simulink model "boat_model_and_controller2020lqi"  (R2021a)
settings: Solver=VariableStepAuto  StartTime=0.0  StopTime=10  FixedStep=0.01  RelTol=1e-3
undefined symbols (not defined in the file): DiscIntNeverNeededParam, Eff, FF_L, FF_R, initial_P, initial_Pitch, initial_Q, initial_R, initial_ROLL, initial_uspeed, initial_vspeed, initial_wspeed, initial_YAW, initial_Z, Kih, Kir, rear_alfas, T, uncertainty
libraries: simulink x7, simulink_extras x3, dspsrcs4 x1, pid_lib x1
(part 2 of 3)

== matlab function boat_model_and_controller2020lqi/BOAT/model_equations ==
  data: u_dot output; v_dot output; w_dot output; p_dot output; q_dot output; r_dot output; Act_front_left input; Act_front_right input; Act_rear input; Rpms_motor input; Rudder input; u input; v input; w input; p input; qq input; r input; Pitch input; Roll input; Yaw input; z input; Torque output; Rpms_motor output; Lift_Coluna output; Lift_Strut_right output; D_total_strut_right output; drag_col output; bb output; kstrut_left output; kcoluna output; uncertainty input
function [u_dot,v_dot,w_dot,p_dot,q_dot,r_dot,Torque,Rpms_motor,Lift_Coluna,Lift_Strut_right,D_total_strut_right,drag_col,bb,kstrut_left,kcoluna] = model_equations(Act_front_left,Act_front_right,Act_rear,Rpms_motor,Rudder,u,v,w,p,qq,r,Pitch,Roll,Yaw,z,uncertainty)

%%%%%%%%%%%%%%%%%%%%%%%%%%%%%%%%%%%%%%%%%%%%%%%%%SS
%%%%%%%%%%%%%%%% constants %%%%%%%%%%%%%%%%%%%%%%
%%%%%%%%%%%%%%%%%%%%%%%%%%%%%%%%%%%%%%%%%%%%%%%%%
pi=3.14159265358979;
g = 9.81; %gravity (m/s^2)
rho= 1025.00; % Densidade de àgua(kg/m^3)   <-I
mu= 1.14E-3; % Coef. Viscosidade Dinâmica para calular Reynolds(Pa*s)   <-I
m = 180*uncertainty(15); %Weight of boat (Kg) <-I
dist_cm_Us_x = 3.150*uncertainty(16);   %distância ultrassom ao cm
dist_struts_Us_x = 1.850*uncertainty(17);
dist_col_Us_x = 5.520*uncertainty(18);
dy_front = 1.2/2*uncertainty(19); %front foils' y distance divided by 2
dist_x_rear = 2.367*uncertainty(20);
dist_x_front = 1.30156*uncertainty(21);
dist_z_rear = 1.05*uncertainty(22); %ambas desde o CM (z também se mede desde o ultrassom)
dist_z_front = 0.85*uncertainty(23);
coluna_exposta = 0.776*uncertainty(24);
z_cm_sem_roll = cosd(Pitch)*z+tand(Pitch)*dist_cm_Us_x;
z_cm = z_cm_sem_roll/cosd(Roll);
z_struts_sem_roll = z+dist_struts_Us_x*tand(Pitch);
z_col_sem_roll = z+dist_col_Us_x*tand(Pitch); %perpendicular à água no roll
z_strut_left = z_struts_sem_roll - tand(Roll)*dy_front;
z_strut_right = z_struts_sem_roll + tand(Roll)*dy_front;
hf_left = dist_z_front +z_strut_left;
hf_right = dist_z_front+z_strut_right;
hr = dist_z_rear + z_col_sem_roll;

if hr > coluna_exposta
    hr = coluna_exposta;
end
if hf_left > dist_z_front
    hf_left = dist_z_front;
end
if hf_right > dist_z_front
    hf_right = dist_z_front;
end
Iyy = 503*uncertainty(11);        % boat's moment of inertia in kg.m^2 for pitch
Ixx = 31*uncertainty(12);          % moment of inertia for roll
Izz = 300*uncertainty(13);
Ixz = 16.5*uncertainty(14);

%angle of attack
aa = atand(w/u);
bb = asind(v/sqrt(u^2+v^2));
alfa_front_left = Act_front_left + aa;
alfa_front_right = Act_front_right + aa;
alfa_rear = Act_rear + aa;
speed = sqrt(u^2+v^2+w^2);

%%%%%%%%%%%%%%%%%%%%%%%%%%%%%%%%%%%%%%%%%%%%%%%%%
%%%%%%%%%%%%%%%% Geometry %%%%%%%%%%%%%%%%%%%%%%%
%%%%%%%%%%%%%%%%%%%%%%%%%%%%%%%%%%%%%%%%%%%%%%%%%
a = 1;
%Geometria foil frente(x2)
cff=0.08; % Corda foil frente(m)
tff=0.12; % Espessura maxima perfil foil frente (n63412: t=0.12c)
bff=0.8; % Envergadura foil frente (m)
Sff=1.05*pi*bff*cff/4*a; %Area planform foil frente (m^2) --  0.04773 valor dos foils atuais
SAff=Sff*2; % Area superficie foil frente (assumir 2x planform area) (m^2)
ARf=bff^2/Sff; %Aspect ratio foil frente
cordfun = @(x) cff.^2 .*(x-(x.^3/(bff/2).^2)/3);
MACf =  2/Sff*(cordfun(bff/2)-cordfun(0));
cff=MACf;
k2f_left = (16*(hf_left/MACf)^2+2)/(16*(hf_left/MACf)^2+1);
k2f_right = (16*(hf_right/MACf)^2+2)/(16*(hf_right/MACf)^2+1);

%Geometria foil trás
cft=0.08; % Corda foil trás (m)
tft=0.12; % Espessura maxima foil tras (n63412: t=0.12c)
bft=0.8; % Envergadura foil tras (m)
Sft=1.05*pi*bft*cft/4*a; %Area planform foil tras (m^2) --- 0.04584 valor dos foils atuais
SAft=Sft*2; % Area superficie foil tras (assumir 2x planform area) (m^2)
ARt=bft^2/Sft; %Aspect ratio foil tras
cordfun = @(x) cft.^2 .*(x-(x.^3/(bft/2).^2)/3);
MACt = 2/Sft*(cordfun(bft/2)-cordfun(0));
cft=MACt;
k2t = (16*(hr/MACt)^2+2)/(16*(hr/MACf)^2+1);
%Geometria Struts
cs= 0.13; % Corda strut (m)
ts=0.12; % Espessura maxima perfil strut (n0012: t=0.12c)
Ss_left=cs*hf_left; %area planform strut (m^2)
SAs_left=2*Ss_left; % Area superficie strut (SOLIDWORKS) (m^2)
substrut_left=hf_left/cs; %aspect ratio da seccao submergida strut
Ss_right=cs*hf_right; %area planform strut (m^2)
SAs_right=2*Ss_right; % Area superficie strut (SOLIDWORKS) (m^2)
substrut_right=hf_right/cs; %aspect ratio da seccao submergida strut


%Geometria Coluna
cc=0.17; % corda coluna (m)
tc=0.18; % Espessura maxima perfil coluna (n0012: t=0.12c)
Sc=cc*hr; %area planform coluna (m^2)
SAc=2*Sc; % Area superficie coluna (m^2)
subcol=hr/cc; %aspect ratio da seccao submergida coluna


%%%%%%%%%%%%%%%%%%%%%%%%%%%%%%%%%%%%%%%%%%%%%%%%%
%%%%%%%%%%%%%%%% pre-calculations %%%%%%%%%%%%%%%
%%%%%%%%%%%%%%%%%%%%%%%%%%%%%%%%%%%%%%%%%%%%%%%%%

q = 0.5*rho*speed^2;%Pressao dinamica (Kg m^-1 s^-2)

Tff=cff*tff; % Thicknes front foil= chord*t
Tft=cft*tft;% Thicknes rear foil= chord*t
Ts=cs*ts; % Thicknes strut= chord*t
Tc=cc*tc;% Thicknes coluna= chord*t

Reff=(rho)*(speed)*(cff)/(mu); %Num Reynolds foil frente
Reft=(rho)*(speed)*(cft)/(mu); %Num Reynold foil tras
Restrut=(rho)*(speed)*(cs)/(mu); %Num Reynolds strut
Recol=(rho)*(speed)*(cc)/(mu); %Num Reynolds coluna

%determining cd of the foils, struts and prop column

%strut pressure drag. Column assumed to have same pressure drag as
%strut

p00 =     0.01162;
p10 =  -7.938e-07;
p01 =  -5.664e-05;
p20 =   0.0001378;
p11 =   3.735e-08;
p02 =   1.241e-07;
p30 =  -1.257e-07;
p21 =   -4.13e-07;
p12 =  -9.269e-11;
p03 =  -1.231e-10;
p40 =   1.604e-06;
p31 =    4.88e-10;
p22 =   4.056e-10;
p13 =   6.432e-14;
p04 =   5.515e-14;
p50 =  -1.201e-09;
p41 =  -1.096e-09;
p32 =   -1.95e-13;
p23 =   -1.04e-13;
p14 =   -1.36e-17;
p05 =   -9.13e-18;

cdpstrut =@(x,y) p00 + p10*x + p01*y + p20*x^2 + p11*x*y + p02*y^2 + p30*x^3 + p21*x^2*y ...
    + p12*x*y^2 + p03*y^3 + p40*x^4 + p31*x^3*y + p22*x^2*y^2 ...
    + p13*x*y^3 + p04*y^4 + p50*x^5 + p41*x^4*y + p32*x^3*y^2 ...
    + p23*x^2*y^3 + p14*x*y^4 + p05*y^5;

CDp_s = cdpstrut(bb,Restrut/1000)*uncertainty(1);
CDp_c = cdpstrut(bb+Rudder,Recol/1000)*uncertainty(2);

%determining coefficient of lift of the foils for a set angle of attack
p00 =     0.04647;
p10 =      0.1369;
p01 =    0.001502;
p20 =   0.0005872;
p11 =  -0.0001138;
p02 =  -2.794e-06;
p30 =  -0.0007229;
p21 =  -2.662e-07;
p12 =   1.545e-07;
p03 =   2.428e-09;
p40 =   1.647e-05;
p31 =   6.574e-07;
p22 =  -3.892e-09;
p13 =  -7.221e-11;
p04 =  -9.966e-13;
p50 =  -6.807e-08;
p41 =  -2.534e-09;
p32 =  -2.657e-10;
p23 =   2.267e-12;
p14 =   9.751e-15;
p05 =   1.555e-16;

clf = @(x,y) p00 + p10*x + p01*y + p20*x^2 + p11*x*y + p02*y^2 + p30*x^3 + p21*x^2*y ...
    + p12*x*y^2 + p03*y^3 + p40*x^4 + p31*x^3*y + p22*x^2*y^2 ...
    + p13*x*y^3 + p04*y^4 + p50*x^5 + p41*x^4*y + p32*x^3*y^2 ...
    + p23*x^2*y^3 + p14*x*y^4 + p05*y^5;

clff_left = clf(alfa_front_left,Reff/1000)*uncertainty(3);
clff_right = clf(alfa_front_right,Reff/1000)*uncertainty(3);
clrf = clf(alfa_rear,Reft/1000)*uncertainty(4);
CL_f_3D_left =clff_left*(ARf/(ARf+2))*k2f_left;
CL_f_3D_right =clff_right*(ARf/(ARf+2))*k2f_right;
CL_t_3D =clrf*(ARt/(ARt+2))*k2t;

%determining coefficient of pressure drag of the foils
p00 =     0.01465;
p10 =  -0.0003439;
p01 =  -5.436e-05;
p20 =  -0.0002518;
p11 =   1.629e-06;
p02 =   8.999e-08;
p30 =   1.962e-05;
p21 =   5.111e-07;
p12 =  -2.115e-09;
p03 =  -7.446e-11;
p40 =    6.85e-06;
p31 =  -4.153e-08;
p22 =  -2.604e-10;
p13 =   1.213e-12;
p04 =   3.002e-14;
p50 =  -3.572e-07;
p41 =  -2.379e-09;
p32 =   1.914e-11;
p23 =   3.918e-14;
p14 =  -2.599e-16;
p05 =  -4.682e-18;

cdpf = @(x,y) p00 + p10*x + p01*y + p20*x^2 + p11*x*y + p02*y^2 + p30*x^3 + p21*x^2*y ...
    + p12*x*y^2 + p03*y^3 + p40*x^4 + p31*x^3*y + p22*x^2*y^2 ...
    + p13*x*y^3 + p04*y^4 + p50*x^5 + p41*x^4*y + p32*x^3*y^2 ...
    + p23*x^2*y^3 + p14*x*y^4 + p05*y^5;

cdp_ff_left = cdpf(alfa_front_left,Reff/1000)*uncertainty(5);
cdp_ff_right = cdpf(alfa_front_right,Reff/1000)*uncertainty(5);
cdp_ft = cdpf(alfa_rear,Reft/1000)*uncertainty(6);

%%%%%%%%%%%%%%%%%%%%%%%%%%%%%%%%%%%%%%%%%%%%%%%%%
%%%%%%%%%%%% boat model equations %%%%%%%%%%%%%%%
%%%%%%%%%%%%%%%%%%%%%%%%%%%%%%%%%%%%%%%%%%%%%%%%%

%Lift (XFRL5)
lift_front_left=(CL_f_3D_left)*q*Sff;
lift_front_right=(CL_f_3D_right)*q*Sff;
lift_rear=(CL_t_3D)*q*Sft;

kstrut_left=1/(13+(13/(substrut_left)^2)+(26/(substrut_left)))*uncertainty(7); % coeficiente de lift que toma em conta a aspect ratio da seccao submergida da strut
kstrut_right=1/(13+(13/(substrut_right)^2)+(26/(substrut_right)))*uncertainty(7); % coeficiente de lift que toma em conta a aspect ratio da seccao submergida da strut
kcoluna=1/(13+(13/(subcol)^2)+(26/(subcol)))*uncertainty(8); % coeficiente de lift que toma em conta a aspect ratio da seccao submergida da coluna
Lift_Strut_left = -1/2*rho*(speed^2)*Ss_left*kstrut_left*bb;
Lift_Strut_right = -1/2*rho*(speed^2)*Ss_right*kstrut_right*bb;
Lift_Coluna = -1/2*rho*(speed^2)*Sc*kcoluna*(bb+Rudder);
bb_Trans_sup = 12;
bb_Trans_inf = 15;

if bb>bb_Trans_sup || bb<-bb_Trans_sup % condicão de ventilacão da strut
    Lift_Strut_Trans_sup_left = -1/2*rho*(speed^2)*Ss_left*kstrut_left*bb_Trans_sup*bb/abs(bb);
    Lift_Strut_Trans_sup_right = -1/2*rho*(speed^2)*Ss_right*kstrut_right*bb_Trans_sup*bb/abs(bb);
    Lift_Strut_Trans_inf_left = -1/2*rho*(speed^2)*Ss_left*(kstrut_left*bb_Trans_inf*bb/abs(bb)-kstrut_left*9*(bb/abs(bb))*abs(1-abs(1/bb_Trans_inf)));
    Lift_Strut_Trans_inf_right = -1/2*rho*(speed^2)*Ss_right*(kstrut_right*bb_Trans_inf*bb/abs(bb)-kstrut_right*9*(bb/abs(bb))*abs(1-abs(1/bb_Trans_inf)));
    Lift_Strut_left = Lift_Strut_Trans_sup_left+(Lift_Strut_Trans_inf_left-Lift_Strut_Trans_sup_left)/(bb_Trans_inf*bb/abs(bb)-bb_Trans_sup*bb/abs(bb))*(bb-bb_Trans_sup*bb/abs(bb));
    Lift_Strut_right = Lift_Strut_Trans_sup_right+(Lift_Strut_Trans_inf_right-Lift_Strut_Trans_sup_right)/(bb_Trans_inf*bb/abs(bb)-bb_Trans_sup*bb/abs(bb))*(bb-bb_Trans_sup*bb/abs(bb));
    if bb>bb_Trans_inf || bb<-bb_Trans_inf
        Lift_Strut_left = -1/2*rho*(speed^2)*Ss_left*(kstrut_left*bb-kstrut_left*9*(bb/abs(bb))*abs(1-abs(1/bb)));
        Lift_Strut_right = -1/2*rho*(speed^2)*Ss_right*(kstrut_right*bb-kstrut_right*9*(bb/abs(bb))*abs(1-abs(1/bb)));
    end
end
if (bb+Rudder)>bb_Trans_sup || (bb+Rudder)<-bb_Trans_sup
    Lift_Coluna = -1/2*rho*speed^2*Sc*(kcoluna*(bb+Rudder)-kcoluna*9*(bb+Rudder)/abs(bb+Rudder));
end

%Induced Drag (XFLR5)
e=1; %oswald efficiency factor (assumir 1 para dist. lift puramente eliptica)
C_Dind_ff_left=(CL_f_3D_left)^2/(pi*e*(ARf)); % Coef Drag Induzido
C_Dind_ff_right=(CL_f_3D_right)^2/(pi*e*(ARf)); % Coef Drag Induzido
C_Dind_rf=(CL_t_3D)^2/(pi*e*(ARt));
D_induced_ff_left=(C_Dind_ff_left)*q*(Sff); %Drag induzido (N)
D_induced_ff_right=(C_Dind_ff_right)*q*(Sff); %Drag induzido (N)
D_induced_rf=(C_Dind_rf)*q*(Sft); %Drag induzido (N)

% Skin Friction Drag

Re_crit=500000;  %Como Rule Of Thumb, assume-se que a transição se dá pontualemente a Re=500 000- Anderson's Fundamentals of Aerodynamics (pg 903)
x_crit=Re_crit*mu/(rho*speed); %calcula o ponto onde se dá a transição na asa retângular
%x_c_crit_n63412=; %  <-M
%x_c_crit_n0012=0.3; %     <-M
%VARIAVEIS DE INPUT VAZIAS PARA FORÇAR A
%TRANSIÇAO NUM PONTO QUE NAO RE 500 000

%Foils frente

C_skf_ff_lam=1.328/(Re_crit)^0.5; %Coef skin friction esc laminar- Hoerner’s Fluid-Dynamic Drag (pg 2-5)-Foil frente
S_ff_lam=Sff*x_crit; %Area de escoamento laminar- corresponde a zona 1-lam
D_skf_ff_lam=q*C_skf_ff_lam*S_ff_lam; %Drag skf foil frente_flat plate_zona 1-lam
C_skf_ff_tur_12=0.455/(log10(Reff)^2.58); %Coef skin friction esc turbulento- Hoerner’s Fluid-Dynamic Drag (pg 2-5)-fim zona 2-tur
C_skf_ff_tur_1=0.455/(log10(Re_crit)^2.58); %coef skf ff esc turbulento- fim zona 1-trans
D_skf_ff_tur_12=q*Sff*C_skf_ff_tur_12; %drag skf ff_flat plate_esc turbulento-fim zona 2-tur
D_skf_ff_tur_1=q*S_ff_lam*C_skf_ff_tur_1;%drag skf ff_flat plate_esc turbulento- fim zona 1-trans
D_skf_ff_tur=D_skf_ff_tur_12-D_skf_ff_tur_1;%drag skf ff_flat plate_esc turbulento total
D_skf_ff_tot_1=D_skf_ff_lam +D_skf_ff_tur; %drag skf ff_flat plate_total
CD_skf_ff=D_skf_ff_tot_1/(q*Sff); %coeficiente de drag de skin friction ff final
D_ffskf=1/2*(CD_skf_ff)*(rho)*(speed)^2*(SAff); %Drag de skin friction final ff


%Foil Tras
C_skf_ft_lam=1.328/(Re_crit)^0.5;%Coef skin friction esc laminar- Hoerner’s Fluid-Dynamic Drag (pg 2-5)-Foil tras
S_ft_lam=Sft*x_crit; %Area de escoamento laminar- corresponde a zona 1-lam
D_skf_ft_lam=q*C_skf_ft_lam*S_ft_lam;%Drag skf foil tras_flat plate_zona 1-lam
C_skf_ft_tur_12=0.455/(log10(Reff)^2.58); %Coef skin friction esc turbulento- Hoerner’s Fluid-Dynamic Drag (pg 2-5)-fim zona 2-tur
C_skf_ft_tur_1=0.455/(log10(Re_crit)^2.58); %coef skf ft esc turbulento- fim zona 1-trans
D_skf_ft_tur_12=q*Sft*C_skf_ft_tur_12;%drag skf ft_flat plate_esc turbulento-fim zona 2-tur
D_skf_ft_tur_1=q*S_ft_lam*C_skf_ft_tur_1;%drag skf ft_flat plate_esc turbulento- fim zona 1-trans
D_skf_ft_tur=D_skf_ft_tur_12-D_skf_ft_tur_1;%drag skf ft_flat plate_esc turbulento total
D_skf_ft_tot_1=D_skf_ft_lam +D_skf_ft_tur; %drag skf ft_flat plate_total
CD_skf_ft=D_skf_ft_tot_1/(q*Sft);%coeficiente de drag de skin friction ft final
D_ftskt=1/2*(CD_skf_ft)*(rho)*(speed)^2*(SAft);%Drag de skin friction final ft



%Strut Esquerda
C_skf_s_lam=1.328/(Re_crit)^0.5;%Coef skin friction esc laminar- Hoerner’s Fluid-Dynamic Drag (pg 2-5)-strut
S_s_lam_left=Ss_left*x_crit; %Area de escoamento laminar- corresponde a zona 1-lam
D_skf_s_lam_left=q*C_skf_s_lam*S_s_lam_left;%Drag skf strut_flat plate_zona 1-lam
C_skf_s_tur_12=0.455/(log10(Restrut)^2.58);%Coef skin friction esc turbulento- Hoerner’s Fluid-Dynamic Drag (pg 2-5)-fim zona 2-tur
C_skf_s_tur_1=0.455/(log10(Re_crit)^2.58);%coef skf s esc turbulento- fim zona 1-trans
D_skf_s_tur_12_left=q*Ss_left*C_skf_s_tur_12;%drag skf s_flat plate_esc turbulento-fim zona 2-tur
D_skf_s_tur_1_left=q*S_s_lam_left*C_skf_s_tur_1;%drag skf s_flat plate_esc turbulento- fim zona 1-trans
D_skf_s_tur_left=D_skf_s_tur_12_left-D_skf_s_tur_1_left; %drag skf s_flat plate_esc turbulento total
D_skf_s_tot_1_left=D_skf_s_lam_left +D_skf_s_tur_left; %drag skf s_flat plate_total
CD_skf_s_left=D_skf_s_tot_1_left/(q*Ss_left);%coeficiente de drag de skin friction s final
D_strutskf_left=1/2*(CD_skf_s_left)*(rho)*(speed)^2*(SAs_left);%Drag de skin friction final strut

%Strut Direita
C_skf_s_lam=1.328/(Re_crit)^0.5;%Coef skin friction esc laminar- Hoerner’s Fluid-Dynamic Drag (pg 2-5)-strut
S_s_lam_right=Ss_right*x_crit; %Area de escoamento laminar- corresponde a zona 1-lam
D_skf_s_lam_right=q*C_skf_s_lam*S_s_lam_right;%Drag skf strut_flat plate_zona 1-lam
C_skf_s_tur_12=0.455/(log10(Restrut)^2.58);%Coef skin friction esc turbulento- Hoerner’s Fluid-Dynamic Drag (pg 2-5)-fim zona 2-tur
C_skf_s_tur_1=0.455/(log10(Re_crit)^2.58);%coef skf s esc turbulento- fim zona 1-trans
D_skf_s_tur_12_right=q*Ss_right*C_skf_s_tur_12;%drag skf s_flat plate_esc turbulento-fim zona 2-tur
D_skf_s_tur_1_right=q*S_s_lam_right*C_skf_s_tur_1;%drag skf s_flat plate_esc turbulento- fim zona 1-trans
D_skf_s_tur_right=D_skf_s_tur_12_right-D_skf_s_tur_1_right; %drag skf s_flat plate_esc turbulento total
D_skf_s_tot_1_right=D_skf_s_lam_right +D_skf_s_tur_right; %drag skf s_flat plate_total
CD_skf_s_right=D_skf_s_tot_1_right/(q*Ss_right);%coeficiente de drag de skin friction s final
D_strutskf_right=1/2*(CD_skf_s_right)*(rho)*(speed)^2*(SAs_right);%Drag de skin friction final strut


%coluna
C_skf_c_lam=1.328/(Re_crit)^0.5;%Coef skin friction esc laminar- Hoerner’s Fluid-Dynamic Drag (pg 2-5)-coluna
S_c_lam=Sc*x_crit;%Area de escoamento laminar- corresponde a zona 1-lam
D_skf_c_lam=q*C_skf_c_lam*S_c_lam;%Drag skf coluna_flat plate_zona 1-lam
C_skf_c_tur_lt=0.455/(log10(Recol)^2.58);%Coef skin friction esc turbulento- Hoerner’s Fluid-Dynamic Drag (pg 2-5)-fim zona 2-tur
C_skf_c_tur_l=0.455/(log10(Re_crit)^2.58);%coef skf c esc turbulento- fim zona 1-trans
D_skf_c_tur_lt=q*Sc*C_skf_c_tur_lt;%drag skf c_flat plate_esc turbulento-fim zona 2-tur
D_skf_c_tur_l=q*S_c_lam*C_skf_c_tur_l;%drag skf c_flat plate_esc turbulento- fim zona 1-trans
D_skf_c_tur=D_skf_c_tur_lt-D_skf_c_tur_l;%drag skf c_flat plate_esc turbulento total
D_skf_c_tot_1=D_skf_c_lam +D_skf_c_tur;%drag skf c_flat plate_total
CD_skf_c=D_skf_c_tot_1/(q*Sc);%coeficiente de drag de skin friction c final
D_skfc=1/2*(CD_skf_c)*(rho)*(speed)^2*(SAc); %Drag de skin friction final coluna

%Form Drag
D_form_ff_left=(cdp_ff_left)*q*(Sff);
D_form_ff_right=(cdp_ff_right)*q*(Sff);
D_form_rf=(cdp_ft)*q*(Sft);
D_form_s_left=(CDp_s)*q*(Ss_left);
D_form_s_right=(CDp_s)*q*(Ss_right);
D_form_c=(CDp_c)*q*(2*Sc);

%Drag de Interferência
C_Dint_ff=17*(tff)^2-.05; %Coef Drag interferencia- Hoerner’s Fluid Dynamic Drag (pg 8-1)
C_Dint_rf=17*(tft)^2-.05; %Coef Drag interferencia- Hoerner’s Fluid Dynamic Drag (pg 8-1)
D_interference_ff=q*(C_Dint_ff)*((Tff+Ts)/2)^2;%Drag Interferencia (N)
D_interference_rf=q*(C_Dint_rf)*((Tft+Tc)/2)^2;%Drag Interferencia (N)

%Spray Drag
F_hs_left= speed/(g*hf_left)^(0.5);%Numero de Froude a profundidade da strut
F_hs_right= speed/(g*hf_right)^(0.5);%Numero de Froude a profundidade da strut
F_hc= speed/(g*hr)^(0.5);%Numero de Froude a profundidade da coluna
%A expressao utilizada de drag de spray aplica se para numeros de
%Froude ~3<
CDs=0.24; %coeficiente empirico de spray @Hoerner_Fluid-Dynamic Drag (10-13)
Ds_s=q*CDs*(ts*cs)^2;%Drag de spray para uma strut
Ds_c=q*CDs*(tc*cc)^2;%Drag de spray para a coluna

%Wave Drag
CDw_s_left=0.5*(CL_f_3D_left/(F_hs_left*2))^2;
CDw_s_right=0.5*(CL_f_3D_right/(F_hs_right*2))^2;
CDw_c=0.5*(CL_t_3D/(F_hc*2))^2;
Dw_ff_left=q*CDw_s_left*hf_left*bff;
Dw_ff_right=q*CDw_s_right*hf_right*bff;
Dw_ft=q*CDw_c*hr*bft;


%Total Drag


D_total_ff_right=D_induced_ff_right+D_ffskf+D_form_ff_right+D_interference_ff+Dw_ff_right;
D_total_ff_left=D_induced_ff_left+D_ffskf+D_form_ff_left+D_interference_ff+Dw_ff_left;
D_total_rf=D_induced_rf+D_ftskt+D_form_rf+D_interference_rf+Dw_ft;
D_total_strut_left=D_strutskf_left+D_form_s_left+Ds_s;
D_total_strut_right=D_strutskf_right+D_form_s_right+Ds_s;
drag_col=D_skfc+D_form_c+Ds_c;
drag_front_left = D_total_ff_left;
drag_front_right = D_total_ff_right;

%Hull
CDh = 0.006*uncertainty(9);% CFD Data
zp = -z_cm*100;
if (zp < 32 + 5/22)
    Hull_area = -0.2167*zp+6.98365;
else
    Hull_area = 0;
end
D_HULL = 0.5*CDh*rho*Hull_area*speed^2;
V_HULL = 0.001*zp^2-0.064*zp+1.03025;
if (zp >= 31)
    V_HULL = 0;
end
BUOYANCY = V_HULL*rho*g;


%calculate Thrust based on rpms
Rpms_helice = Rpms_motor/2.85;
diam = 0.25;

%Interpolation coefficients of thrust
p1 =     -0.2264;
p2 =      0.8165;
p3 =     -0.9315;
p4 =      0.2713;
p5 =   -0.009195;
p6 =   -0.005493;
p7 =      0.1617;

%Interpolation coefficients of proppeler's efficiency

k1 =      -170.6;
k2 =       30.69;
k3 =      -50.99;
k4 =       440.2;
k5 =      -1.744;
q1 =      -201.3;
q2 =       93.96;
q3 =       150.8;
q4 =      -151.9;
q5 =       398.2;

js = 60*speed/(Rpms_helice*diam);
ktfun = @(x) p1*x.^6 + p2*x.^5 + p3*x.^4 + p4*x.^3 + p5*x.^2 + p6*x + p7;

kt =ktfun(js)*uncertainty(10)  ;

Efffun = @(x)(k1*x.^4 + k2*x.^3 + k3*x.^2 + k4*x + k5) /...
    (x.^5 + q1*x.^4 + q2*x.^3 + q3*x.^2 + q4*x + q5);

Eff = Efffun(js);

thrust = rho*(Rpms_helice/60)^2*diam^4*kt;
P_helice = thrust*speed/Eff;

%Calculate Power usage
P_mec=P_helice/0.96;
Torque=P_mec/(Rpms_motor*2*pi/60);

%%%%%%%%%%%%%%%%%%%%%%%%%Balances of forces and momenta%%%%%%%%%%%%%%%%
%%%%%%%%%%%%%%%%%%%%%%%%%%%%%%%%%%%%%%%%%%%%%%%%%%%%%%%%%%%%%%%%%%%%%%%

%Inertial to body frame matrix
R = [cosd(Pitch)*cosd(Yaw) cosd(Pitch)*sind(Yaw) -sind(Pitch);
    sind(Roll)*sind(Pitch)*cosd(Yaw)-cosd(Roll)*sind(Yaw) sind(Roll)*sind(Pitch)*sind(Yaw)+cosd(Roll)*cosd(Yaw) sind(Roll)*cosd(Pitch);
    cosd(Roll)*sind(Pitch)*cosd(Yaw)+sind(Roll)*sind(Yaw) cosd(Roll)*sind(Pitch)*sind(Yaw)-sind(Roll)*cosd(Yaw) cosd(Roll)*cosd(Pitch)];

%Inertial forces
W_inertial = m*g*[0;0;1];
BUOY_inertial = BUOYANCY*[0;0;-1];

%Body frame forces
L_RF = lift_front_right*[sind(aa);0;-cosd(aa)];
L_LF = lift_front_left*[sind(aa);0;-cosd(aa)];
L_RE = lift_rear*[sind(aa);0;-cosd(aa)];
D_RE = D_total_rf*[-cosd(aa);0;-sind(aa)];
D_RF = drag_front_right*[-cosd(aa);0;-sind(aa)];
D_LF = drag_front_left*[-cosd(aa);0;-sind(aa)];
D_HU = D_HULL*[-u/speed;-v/speed;-w/speed];
W    = R*W_inertial;
BUOY = R*BUOY_inertial;
% Lift_Strut_left  = -1/2*rho*(speed)^2*Ss_left*0.1121*bb;
% Lift_Strut_right  = -1/2*rho*(speed)^2*Ss_right*0.1121*bb;
% Lift_Coluna  = -1/2*rho*(speed^2)*Sc*0.1121*(bb+Rudder);
%Sum of body frame forces in each location to calculate momenta
X_LF = L_LF(1)+D_LF(1);
Y_LF = 0;
Z_LF = L_LF(3)+D_LF(3);
X_LS = -Lift_Strut_left*sind(bb)-D_total_strut_left*cosd(bb);
Y_LS = Lift_Strut_left*cosd(bb)-D_total_strut_left*sind(bb);
Z_LS = 0;
X_RF = L_RF(1)+D_RF(1);
Y_RF = 0;
Z_RF = L_RF(3)+D_RF(3);
X_RS = -Lift_Strut_right*sind(bb)-D_total_strut_right*cosd(bb);
Y_RS = Lift_Strut_right*cosd(bb)-D_total_strut_right*sind(bb);
Z_RS = 0;
X_RE = L_RE(1)+D_RE(1);
Y_RE =  0;
Z_RE = L_RE(3)+D_RE(3);
X_Col = -Lift_Coluna*sind(bb)-drag_col*cosd(bb);
Y_Col =  Lift_Coluna*cosd(bb)-drag_col*sind(bb);
Z_Col = 0;
Y_Hel = -thrust*sind(Rudder);
X_Hel = thrust*cosd(Rudder);

%Sum of body forces in body axis
X = X_LF + X_RF + X_RE + X_LS + X_RS + X_Col + X_Hel + W(1) + BUOY(1) + D_HU(1);
Y = Y_LF + Y_RF + Y_RE + Y_LS + Y_RS + Y_Col + Y_Hel + W(2) + BUOY(2) + D_HU(2);
Z = Z_LF + Z_RF + Z_RE + Z_LS + Z_RS + Z_Col + W(3) + BUOY(3)+ D_HU(3);

%strut and column lift center depende on heave
dist_z_coluna = hr/2 - z_col_sem_roll; 
dist_z_strut_left = hf_left/2 - z_strut_left;
dist_z_strut_right = hf_right/2 - z_strut_right;

%Sum of moments in body axis
L = -Y_LS*dist_z_strut_left-Z_LF*dy_front-Y_RS*dist_z_strut_right +Z_RF*dy_front-Y_Col*dist_z_coluna - Y_Hel*(dist_z_rear-0.2);
M = X_LF*dist_z_front+X_LS*dist_z_strut_left + X_RF*dist_z_front+X_RS*dist_z_strut_right-Z_LF*dist_x_front-Z_RF*dist_x_front+Z_RE*dist_x_rear+X_RE*dist_z_rear+X_Col*dist_z_coluna+X_Hel*(dist_z_front);
N = X_LF*dy_front+X_LS*dy_front-X_RF*dy_front-X_RS*dy_front+Y_LF*dist_x_front+Y_LS*dist_x_front+Y_RF*dist_x_front+Y_RS*dist_x_front-Y_RE*dist_x_rear-Y_Col*dist_x_rear-Y_Hel*dist_x_rear;

%Balance of forces
r = r*pi/180;
p = p*pi/180;
qq = qq*pi/180;
u_dot = X/m-qq*w+r*v;
v_dot = Y/m+p*w-u*r;
w_dot = Z/m-p*v+qq*u;

%Balance of moments
p_dot = (L/Ixx+Ixz*N/(Ixx*Izz)-Ixz^2/(Ixx*Izz)*qq*r+Ixz/Ixx*(1+(Ixx-Iyy)/Izz)*p*qq+(Iyy-Izz)/Ixx*qq*r)/(1-Ixz^2/(Ixx*Izz));
r_dot = N/Izz+Ixz/Izz*(p_dot-qq*r)+(Ixx-Iyy)/Izz*p*qq;
q_dot = M/Iyy+Ixz/Iyy*(r^2-p^2)+(Izz-Ixx)/Iyy*r*p;
p_dot = p_dot*180/pi;
q_dot = q_dot*180/pi;
r_dot = r_dot*180/pi;
end

== matlab function boat_model_and_controller2020lqi/Controller/LQI_roll1/Gain scheduling1 ==
  data: Kr input; Kr_s output; v input
function Kr_s = fcn(Kr,v)
v_ref = 7;
if(v>v_ref)
    Kr_s = Kr*v_ref/v;
else
    Kr_s = Kr;
end

== matlab function boat_model_and_controller2020lqi/BOAT/Power Consumption Block/MATLAB Function1 ==
  data: Torque input; P_elec output; Rpms_motor input; Eficiencia_motor input
function P_elec = fcn(Torque,Rpms_motor,Eficiencia_motor)
P_mec = Torque*Rpms_motor*2*pi/60;
P_elec = P_mec/Eficiencia_motor;

== matlab function boat_model_and_controller2020lqi/BOAT1/Power Consumption Block/MATLAB Function1 ==
  data: Torque input; P_elec output; Rpms_motor input; Eficiencia_motor input
function P_elec = fcn(Torque,Rpms_motor,Eficiencia_motor)
P_mec = Torque*Rpms_motor*2*pi/60;
P_elec = P_mec/Eficiencia_motor;
